simulink model "EngDa_tiEngOn"  (R2016b)
settings: configuration reference "CodeGenConfigSet" (kept outside this file)
undefined symbols (not defined in the file or in its folder): EngDa_tiEngOn_DT, EngState_conv
libraries: CXLib x1
settings Model: Creator=lenovo  LastModifiedBy=zhoutinglin
settings ConfigSetRef: SourceLocation=Base Workspace

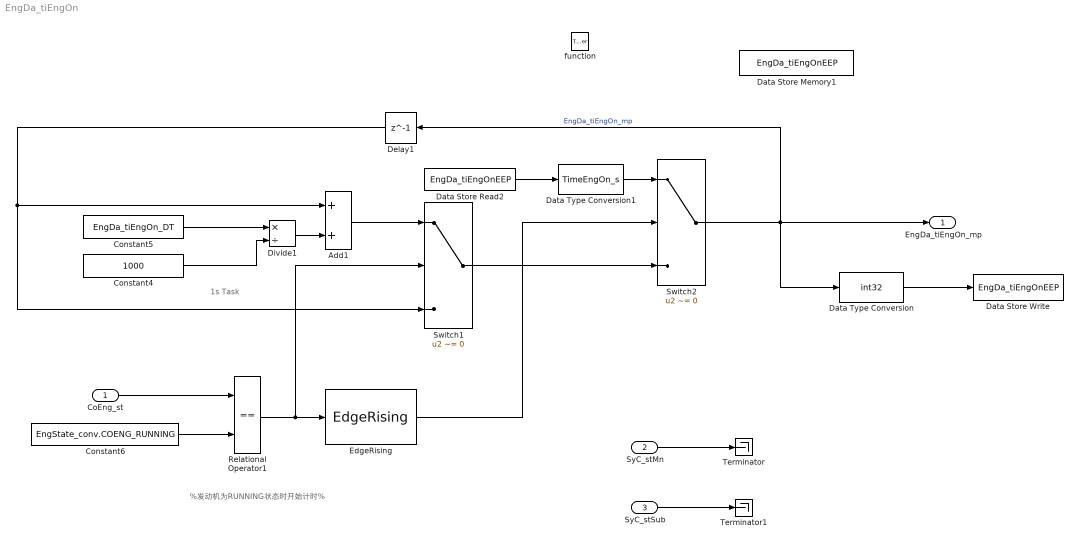
== system EngDa_tiEngOn ==
  note: 1s Task
  note: %发动机为RUNNING状态时开始计时%
  CoEng_st : Inport  Description=Engine coordinator state  OutDataTypeStr=Enum: EngState_conv
  SyC_stMn : Inport  Description=Current system/ECU state  Port=2  OutDataTypeStr=Enum: SysExeState_conv
  SyC_stSub : Inport  Description=Current system/ECU sub-state  Port=3  OutDataTypeStr=Enum: SubSysExeState_conv
  function : TriggerPort  TriggerType=function-call  VariantControl=Variant
  Add1 : Sum  SaturateOnIntegerOverflow=on  InputSameDT=on
  Constant4 : Constant  Value=1000  OutDataTypeStr=uint16
  Constant5 : Constant  Value=EngDa_tiEngOn_DT
  Constant6 : Constant  Value=EngState_conv.COENG_RUNNING
  Data Store Memory1 : DataStoreMemory  DataStoreName=EngDa_tiEngOnEEP  ReadBeforeWriteMsg=warning  WriteAfterWriteMsg=warning  WriteAfterReadMsg=warning  ShowAdditionalParam=off  OutDataTypeStr=int32
  Data Store Read2 : DataStoreRead  DataStoreName=EngDa_tiEngOnEEP
  Data Store Write : DataStoreWrite  DataStoreName=EngDa_tiEngOnEEP
  Data Type Conversion : DataTypeConversion  OutDataTypeStr=int32
  Data Type Conversion1 : DataTypeConversion  OutDataTypeStr=TimeEngOn_s
  Delay1 : Delay  DelayLength=1  InitialCondition=0
  Divide1 : Product  Inputs=*/  OutDataTypeStr=TimeEngOn_s  SaturateOnIntegerOverflow=on
  EdgeRising : CXLib/EdgeRising
  Relational Operator1 : RelationalOperator  Operator===  OutDataTypeStr=boolean  RndMeth=Simplest
  Switch1 : Switch  Criteria=u2 ~= 0  InputSameDT=on
  Switch2 : Switch  Criteria=u2 ~= 0  OutDataTypeStr=Inherit: Inherit via back propagation  InputSameDT=on
  Terminator : Terminator
  Terminator1 : Terminator
  EngDa_tiEngOn_mp : Outport  Tag=s  Description=Engine on time  OutMin=-2147483648  OutMax=2147483647  OutDataTypeStr=TimeEngOn_s
  wires:
  SyC_stSub/1 -> Terminator1/1
  SyC_stMn/1 -> Terminator/1
  CoEng_st/1 -> Relational Operator1/1
  Constant6/1 -> Relational Operator1/2
  Switch2/1 -> Data Type Conversion/1, EngDa_tiEngOn_mp/1, Delay1/1  "EngDa_tiEngOn_mp"
  Delay1/1 -> Add1/1, Switch1/3
  Relational Operator1/1 -> Switch1/2, EdgeRising/1
  Switch1/1 -> Switch2/3
  EdgeRising/1 -> Switch2/2
  Add1/1 -> Switch1/1
  Divide1/1 -> Add1/2
  Constant5/1 -> Divide1/1
  Constant4/1 -> Divide1/2
  Data Store Read2/1 -> Data Type Conversion1/1
  Data Type Conversion/1 -> Data Store Write/1
  Data Type Conversion1/1 -> Switch2/1
